simulink model "power_microgrid_LTE_DR"  (R2017b)
settings: Solver=ode23tb  StartTime=0.0  StopTime=7.5  FixedStep=1/(1000)  MaxStep=60  RelTol=1e-4
PreLoadFcn:
  | load('solar_load_data_24h.mat')
values from neighbouring files (symbols this model uses):
  HPD_1min = [1086.95652174 1079.71014493 1072.46376812 1065.2173913 1057.97101449 1050.72463768 1043.47826087 1036.23188406 1028.98550725 1021.73913043 1014.49275362 1007.24637681 ... (1441 elements, 1441x1)]    [HBD_1min.mat]
  HPT_1min = [0.01 0.02 0.03 0.04 0.05 0.06 0.07 0.08 0.09 0.1 0.11 0.12 ... (1441 elements, 1441x1)]    [HPT_1min.mat]    (also in MainTest.m = (0:7.5/1440:7.5)')
  SPD_1min = [0 0 0 0 0 0 0 0 0 0 0 0 ... (1441 elements, 1441x1)]    [SBD_1min.mat]
  SPT_1min = (0:7.5/1440:7.5)'    [MainTest.m]    (also in SPT_1min.mat = [0 60 120 180 240 300 360 420 480 540 600 660 ... (1441 elem)
undefined symbols (not defined in the file or in its folder): advanceLTEsim, advanceLTEsimulator, appLayer, entity, toAppLayer
libraries: powerlib x27
Description:
  | Copyright 2008-2017 The MathWorks, Inc.
settings Model: ModifiedByFormat=SPS  ExtModeTrigMode=oneshot  ExtModeArmWhenConnect=off  Creator=MathWorks  LastModifiedBy=SPS
settings SolverCC: InitialStep=1e-4  ZeroCrossAlgorithm=Adaptive
settings DataIOCC: SaveFormat=Array  SignalLoggingSaveFormat=ModelDataLogs  SaveOutput=off  SaveTime=off  SignalLoggingName=sigsOut
settings OptimizationCC: BooleanDataType=off  ExpressionDepthLimit=2147483647  InitFltsAndDblsToZero=on  LifeSpan=inf
settings DebuggingCC: AlgebraicLoopMsg=none  SaveWithParameterizedLinksMsg=none  UnderspecifiedInitializationDetection=Classic  MergeDetectMultiDrivingBlocksExec=none  SignalResolutionControl=TryResolveAllWithWarning  MultiTaskDSMMsg=warning  MultiTaskCondExecSysMsg=none  FcnCallInpInsideContextMsg=warning  AllowSymbolicDim=off  StateNameClashWarn=warning  SFUnexpectedBacktrackingDiag=warning  SFNoUnconditionalDefaultTransitionDiag=warning  SFExecutionAtInitializationDiag=none
settings HardwareCC: ProdBitPerPointer=32  ProdBitPerSizeT=32  ProdBitPerPtrDiffT=32  ProdLargestAtomicFloat=None  ProdIntDivRoundTo=Undefined  ProdEndianess=Unspecified  ProdWordSize=32  ProdHWDeviceType=32-bit Generic  TargetUnknown=on
settings ModelReferenceCC: PropagateSignalLabelsOutOfModel=off
settings RTWCC: Description=Generic Real-Time Target
settings CodeAppCC: StateflowObjectComments=on
settings GRTTargetCC: TargetFcnLib=ansi_tfl_tmw.mat  TargetLangStandard=C89/C90 (ANSI)  GeneratePreprocessorConditionals=Disable all  CombineOutputUpdateFcns=off  GRTInterface=on
settings ConfigComp: CovMetricSettings=dw  CovHtmlReporting=on  CovSaveCumulativeToWorkspaceVar=on  CovSaveSingleToWorkspaceVar=on  CovExternalEMLEnable=off  CovSFcnEnable=off
settings SimscapeCC: SimscapeNormalizeSystem=off

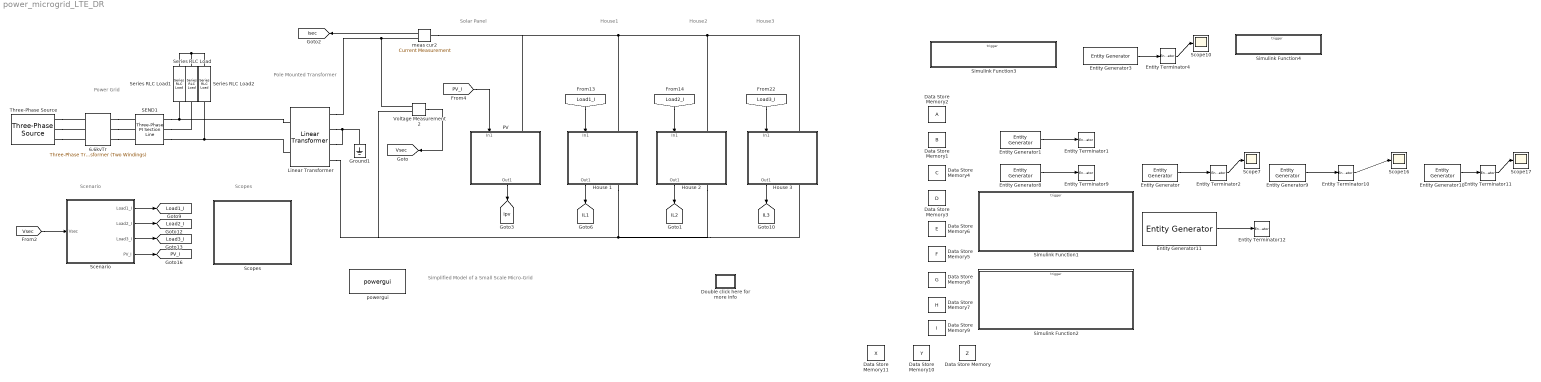
== system power_microgrid_LTE_DR ==
  note: Power Grid
  note: Pole Mounted
      | Transformer
  note: Solar Panel
  note: House1
  note: House2
  note: House3
  note: Scenario
  note: Scopes
  note: Simplified Model of a Small Scale Micro-Grid
  6.6kvTr : powerlib/Elements/Three-Phase Transformer (Two Windings)  Winding1Connection=Yg  Winding2Connection=Y  CoreType=Three single-phase transformers  SetSaturation=off  Hysteresis=off  DataFile='hysteresis'  SetInitialFlux=off  Measurements=None  UNITS=pu  NominalPower=[ 10e6 , 60 ]  Winding1=[ 66e3 , 0.002 , 0.08 ]  Winding2=[6.6e3 , 0.002 , 0.08 ]  Rm=500  Lm=500  L0=0.5  Saturation=[ 0,0 ; 0.0024,1.2 ; 1.0,1.52 ]  InitialFluxes=[ 0.8 , -0.8 , 0.7 ]  MoreParameters=off  BreakLoop=on  DataType=off  TransfoNumber=1
  Data Store Memory : DataStoreMemory  DataStoreName=Z  ReadBeforeWriteMsg=warning  WriteAfterWriteMsg=warning  WriteAfterReadMsg=warning  ShowAdditionalParam=off
  Data Store Memory1 : DataStoreMemory  DataStoreName=B  ReadBeforeWriteMsg=warning  WriteAfterWriteMsg=warning  WriteAfterReadMsg=warning  ShowAdditionalParam=off
  Data Store Memory10 : DataStoreMemory  DataStoreName=Y  ReadBeforeWriteMsg=warning  WriteAfterWriteMsg=warning  WriteAfterReadMsg=warning  ShowAdditionalParam=off
  Data Store Memory11 : DataStoreMemory  DataStoreName=X  ReadBeforeWriteMsg=warning  WriteAfterWriteMsg=warning  WriteAfterReadMsg=warning  ShowAdditionalParam=off
  Data Store Memory2 : DataStoreMemory  ReadBeforeWriteMsg=warning  WriteAfterWriteMsg=warning  WriteAfterReadMsg=warning  ShowAdditionalParam=off
  Data Store Memory3 : DataStoreMemory  DataStoreName=D  ReadBeforeWriteMsg=warning  WriteAfterWriteMsg=warning  WriteAfterReadMsg=warning  ShowAdditionalParam=off
  Data Store Memory4 : DataStoreMemory  DataStoreName=C  ReadBeforeWriteMsg=warning  WriteAfterWriteMsg=warning  WriteAfterReadMsg=warning  ShowAdditionalParam=off
  Data Store Memory5 : DataStoreMemory  DataStoreName=F  ReadBeforeWriteMsg=warning  WriteAfterWriteMsg=warning  WriteAfterReadMsg=warning  ShowAdditionalParam=off
  Data Store Memory6 : DataStoreMemory  DataStoreName=E  ReadBeforeWriteMsg=warning  WriteAfterWriteMsg=warning  WriteAfterReadMsg=warning  ShowAdditionalParam=off
  Data Store Memory7 : DataStoreMemory  DataStoreName=H  ReadBeforeWriteMsg=warning  WriteAfterWriteMsg=warning  WriteAfterReadMsg=warning  ShowAdditionalParam=off
  Data Store Memory8 : DataStoreMemory  DataStoreName=G  ReadBeforeWriteMsg=warning  WriteAfterWriteMsg=warning  WriteAfterReadMsg=warning  ShowAdditionalParam=off
  Data Store Memory9 : DataStoreMemory  DataStoreName=I  ReadBeforeWriteMsg=warning  WriteAfterWriteMsg=warning  WriteAfterReadMsg=warning  ShowAdditionalParam=off
  Double click here for more info : Subsystem
      settings: OpenFcn=showdemo(bdroot(gcb))
      mask Display: disp('?')
  Entity Generator : EntityGenerator  OutputPortMessageModes=m  Period=0.02  GenerateAction=|  AttributeName=nodeID|eventID|Demand  AttributeInitialValue=2|1|1  EntityType=Structured  EntityTypeName=LoadReport1
      | entity.Demand = ReadP();
      | toAppLayer(entity.nodeID,entity.eventID,entity.Demand,0);
  Entity Generator1 : EntityGenerator  OutputPortMessageModes=m  TimeSource=MATLAB action  IntergenerationTimeAction=dt = 0.02; %betarnd(4,4);  GenerateAction=toAppLayer(entity.NodeID,entity.eventID,0,0)  AttributeName=NodeID|eventID  AttributeInitialValue=7|1  EntityType=Structured  EntityTypeName=Forecast
  Entity Generator10 : EntityGenerator  OutputPortMessageModes=m  Period=0.02  GenerateAction=|  AttributeName=nodeID|eventID|Demand  AttributeInitialValue=4|1|1  EntityType=Structured  EntityTypeName=LoadReport3
      | entity.Demand = ReadP();
      | toAppLayer(entity.nodeID,entity.eventID,entity.Demand,0);
  Entity Generator11 : EntityGenerator  OutputPortMessageModes=m  Period=0.02  GenerateAction=|  AttributeName=nodeID|eventID|Psecondary  AttributeInitialValue=1|3|1  EntityType=Structured  EntityTypeName=PriceUpdate_SSPreading
      | entity.Psecondary = ReadPss();
      | toAppLayer(entity.nodeID,entity.eventID,entity.Psecondary,0);
  Entity Generator3 : EntityGenerator  OutputPortMessageModes=m  Period=0.001  GenerateEntityAtSimulationStart=off  GenerateAction=advanceLTEsimulator(entity.data)  AttributeName=data  EntityType=Structured  EntityTypeName=TTIadvance
  Entity Generator8 : EntityGenerator  OutputPortMessageModes=m  TimeSource=MATLAB action  IntergenerationTimeAction=dt = 0.016; %betarnd(4,4);  GenerateAction=toAppLayer(entity.NodeID,entity.eventID,0,0);  AttributeName=NodeID|eventID|phase  AttributeInitialValue=5|1|0  EntityType=Structured  EntityTypeName=PhaseReport
  Entity Generator9 : EntityGenerator  OutputPortMessageModes=m  Period=0.02  GenerateAction=|  AttributeName=nodeID|eventID|Demand  AttributeInitialValue=3|1|1  EntityType=Structured  EntityTypeName=LoadReport2
      | entity.Demand = ReadP();
      | toAppLayer(entity.nodeID,entity.eventID,entity.Demand,0);
  Entity Terminator1 : EntityTerminator  InputPortMessageModes=m
  Entity Terminator{2,4,10..11} (4 alike) : EntityTerminator  InputPortMessageModes=m  NumberEntitiesArrived=on
      settings: OutputPortMap=o0
  Entity Terminator12 : EntityTerminator  InputPortMessageModes=m
  Entity Terminator9 : EntityTerminator  InputPortMessageModes=m
  Ground1 : powerlib/Elements/Ground  LConnTagsString=a
  House 1 : Subsystem
      mask Display: image(imread('house.jpg'))
  House 2 : Subsystem
      mask Display: image(imread('house.jpg'))
  House 3 : Subsystem
      mask Display: image(imread('house.jpg'))
  Linear Transformer : powerlib/Elements/Linear Transformer  UNITS=pu  NominalPower=[75e3 60]  winding1=[ 6600 0.00005 0.0002 ]  winding2=[ 100 0.00005 0.0002 ]  ThreeWindings=on  winding3=[ 100 0.00005 0.0002 ]  RmLm=[ 50 50 ]  Measurements=None  DataType=off
  PV : Subsystem
      mask Display: image(imread('pv.jpg'))
  SEND1 : powerlib/Elements/Three-Phase PI Section Line  LConnTagsString=a|b|c  RConnTagsString=A|B|C  Frequency=60  Resistances=[ 0.01273 0.3864]  Inductances="[ 0.9337e-3  4.1264e-3]"  Capacitances=[12.74e-9 7.751e-9]  Length=1
      settings: SourceProductName=Simscape Power Systems
  Scenario : Subsystem
  Scope{7,10,16..17} (4 alike) : Scope
  Scopes : Subsystem
  Series RLC Load : powerlib/Elements/Series RLC Load  LConnTagsString=a  RConnTagsString=__new0  NominalVoltage=1000  NominalFrequency=60  ActivePower=10e3  InductivePower=100  CapacitivePower=100  Setx0=off  InitialVoltage=0  SetiL0=off  InitialCurrent=0  Measurements=None  LoadType=constant Z
  Series RLC Load1 : powerlib/Elements/Series RLC Load  LConnTagsString=a  RConnTagsString=__new0  NominalVoltage=1000  NominalFrequency=60  ActivePower=100e3  InductivePower=100  CapacitivePower=100  Setx0=off  InitialVoltage=0  SetiL0=off  InitialCurrent=0  Measurements=None  LoadType=constant Z
  Series RLC Load2 : powerlib/Elements/Series RLC Load  LConnTagsString=a  RConnTagsString=__new0  NominalVoltage=1000  NominalFrequency=60  ActivePower=10e3  InductivePower=100  CapacitivePower=100  Setx0=off  InitialVoltage=0  SetiL0=off  InitialCurrent=0  Measurements=None  LoadType=constant Z
  Simulink Function1 : Subsystem  TreatAsAtomicUnit=on
  Simulink Function2 : Subsystem  TreatAsAtomicUnit=on
  Simulink Function3 : Subsystem  TreatAsAtomicUnit=on
  Simulink Function4 : Subsystem  TreatAsAtomicUnit=on
  Three-Phase Source : powerlib/Electrical Sources/Three-Phase Source  InternalConnection=Yg  VoltagePhases=off  Voltage=66e3  PhaseAngle=0  Voltage_phases=[25e3 25e3 25e3]/sqrt(3)  PhaseAngles_phases=[0 -120 +120]  Frequency=60  NonIdealSource=on  SpecifyImpedance=on  Resistance=0.8929  Inductance=16.58e-3  ShortCircuitLevel=100e6  BaseVoltage=25e3  XRratio=7  BusType=swing  Pref=0  Qref=0  Prefabc=[10e3, 10e3, 10e3]  Qrefabc=[0, 0, 0]  Qmin=-inf  Qmax=inf
  Voltage Measurement2 : powerlib/Measurements/Voltage Measurement  PhasorSimulation=on  OutputType=Complex  PSBequivalent=0
  meas cur2 : powerlib/Measurements/Current Measurement  PhasorSimulation=on  OutputType=Complex  PSBequivalent=0
  powergui : powerlib/powergui  SimulationMode=Phasor  SampleTime=1/60/100  frequency=60  Iterations=50  frequencyindice=60  Pbase=100e6  ErrMax=1e-4  UnitsV=kV  UnitsW=MW  buscounter=0  FunctionMessages=off  echomessages=off  EnableUseOfTLC=off  CurrentSourceSwitches=off  DisableSnubberDevices=off  DisableRonSwitches=off  DisableVfSwitches=off  DisplayEquations=off  SolverType=Tustin  Interpol=off  ExternalGateDelay=off  methode=off  Ts=0  x0status=blocks  SPID=off  SwTol=0  HookPort=off  RestoreLinks=warning  ResistiveCurrentMeasurement=off  Frange=[0:2:500]  Ylog=off  Xlog=on  ShowGrid=off  save=off  variable=ZData  structure=0  ZoomFFT=on  StartTime=0.0  cycles=1  DisplayStyle=1  fundamental=60  FreqAxis=off  MaxFrequency=1000  frequencyindicesteady=1  RmsSteady=1  display=off
  tag scope: IL1=global, IL2=global, IL3=global, Ipv=global, Isec=global, Load1_I=global, Load2_I=global, Load3_I=global, PV_I=global, Vsec=global
  wires:
  House 2/1(Out1) -> [IL2]
  House 1/1(Out1) -> [IL1]
  House 3/1(Out1) -> [IL3]
  [Load2_I] -> House 2/1(In1)
  [Load3_I] -> House 3/1(In1)
  PV/1(Out1) -> [Ipv]
  [Vsec] -> Scenario/1(Vsec)
  [Load1_I] -> House 1/1(In1)
  [PV_I] -> PV/1(In1)
  Entity Terminator4/1 -> Scope10/1
  Voltage Measurement2/1 -> [Vsec]
  meas cur2/1 -> [Isec]
  Entity Terminator2/1 -> Scope7/1
  Entity Terminator10/1 -> Scope16/1
  Entity Terminator11/1 -> Scope17/1
  Scenario/4(PV_I) -> [PV_I]
  Scenario/3(Load3_I) -> [Load3_I]
  Scenario/2(Load2_I) -> [Load2_I]
  Scenario/1(Load1_I) -> [Load1_I]
  Entity Generator11/1 -> Entity Terminator12/1
  Entity Generator/1 -> Entity Terminator2/1
  Entity Generator8/1 -> Entity Terminator9/1
  Entity Generator9/1 -> Entity Terminator10/1
  Entity Generator10/1 -> Entity Terminator11/1
  Entity Generator3/1 -> Entity Terminator4/1
  Entity Generator1/1 -> Entity Terminator1/1
  connections:
  SEND1/RConn3 -- Linear Transformer/LConn2 -- Series RLC Load2/RConn1
  6.6kvTr/RConn2 -- SEND1/LConn2
  6.6kvTr/RConn1 -- SEND1/LConn1
  Three-Phase Source/RConn1 -- 6.6kvTr/LConn1
  Three-Phase Source/RConn3 -- 6.6kvTr/LConn3
  6.6kvTr/RConn3 -- SEND1/LConn3
  Ground1/LConn1 -- Linear Transformer/RConn3 -- Linear Transformer/RConn2
  Three-Phase Source/RConn2 -- 6.6kvTr/LConn2
  SEND1/RConn2 -- Series RLC Load/RConn1
  Series RLC Load1/LConn1 -- Series RLC Load/LConn1 -- Series RLC Load2/LConn1
  SEND1/RConn1 -- Linear Transformer/LConn1 -- Series RLC Load1/RConn1
  Linear Transformer/RConn1 -- Voltage Measurement2/LConn1 -- meas cur2/RConn1
  House 2/RConn1 -- House 3/RConn1 -- Linear Transformer/RConn4 -- Voltage Measurement2/LConn2 -- House 1/RConn1
  House 1/LConn1 -- PV/LConn1 -- meas cur2/LConn1 -- House 2/LConn1 -- House 3/LConn1

== system power_microgrid_LTE_DR/Double click here for more info ==

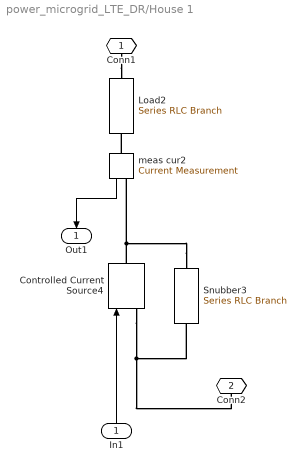
== system power_microgrid_LTE_DR/House 1 ==
  In1 : Inport
  Controlled Current Source4 : powerlib/Electrical Sources/Controlled Current Source  Initialize=on  Source_Type=AC  Amplitude=0  Phase=30  Frequency=60  Measurements=None
  Load2 : powerlib/Elements/Series RLC Branch  LConnTagsString=__new0  RConnTagsString=__new0  BranchType=R  Resistance=16  Inductance=1e-3  SetiL0=off  InitialCurrent=0  Capacitance=1e-6  Setx0=off  InitialVoltage=0  Measurements=None
  Snubber3 : powerlib/Elements/Series RLC Branch  LConnTagsString=__new0  RConnTagsString=__new0  BranchType=R  Resistance=1e6  Inductance=1e-3  SetiL0=off  InitialCurrent=0  Capacitance=1e-6  Setx0=off  InitialVoltage=0  Measurements=None
  meas cur2 : powerlib/Measurements/Current Measurement  PhasorSimulation=on  OutputType=Complex  PSBequivalent=0
  Conn1 : PMIOPort  Port=1  Side=Left
  Conn2 : PMIOPort  Port=2  Side=Right
  Out1 : Outport
  wires:
  In1/1 -> Controlled Current Source4/1
  meas cur2/1 -> Out1/1
  connections:
  Conn1/RConn1 -- Load2/LConn1
  meas cur2/LConn1 -- Load2/RConn1
  Snubber3/LConn1 -- meas cur2/RConn1 -- Controlled Current Source4/RConn1
  Snubber3/RConn1 -- Conn2/RConn1 -- Controlled Current Source4/LConn1

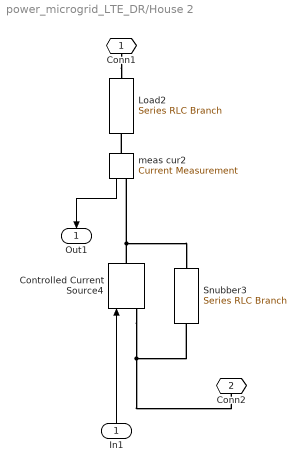
== system power_microgrid_LTE_DR/House 2 ==
  In1 : Inport
  Controlled Current Source4 : powerlib/Electrical Sources/Controlled Current Source  Initialize=on  Source_Type=AC  Amplitude=0  Phase=30  Frequency=60  Measurements=None
  Load2 : powerlib/Elements/Series RLC Branch  LConnTagsString=__new0  RConnTagsString=__new0  BranchType=R  Resistance=16  Inductance=1e-3  SetiL0=off  InitialCurrent=0  Capacitance=1e-6  Setx0=off  InitialVoltage=0  Measurements=None
  Snubber3 : powerlib/Elements/Series RLC Branch  LConnTagsString=__new0  RConnTagsString=__new0  BranchType=R  Resistance=1e6  Inductance=1e-3  SetiL0=off  InitialCurrent=0  Capacitance=1e-6  Setx0=off  InitialVoltage=0  Measurements=None
  meas cur2 : powerlib/Measurements/Current Measurement  PhasorSimulation=on  OutputType=Complex  PSBequivalent=0
  Conn1 : PMIOPort  Port=1  Side=Left
  Conn2 : PMIOPort  Port=2  Side=Right
  Out1 : Outport
  wires:
  meas cur2/1 -> Out1/1
  In1/1 -> Controlled Current Source4/1
  connections:
  Controlled Current Source4/LConn1 -- Conn2/RConn1 -- Snubber3/RConn1
  Controlled Current Source4/RConn1 -- meas cur2/RConn1 -- Snubber3/LConn1
  meas cur2/LConn1 -- Load2/RConn1
  Conn1/RConn1 -- Load2/LConn1

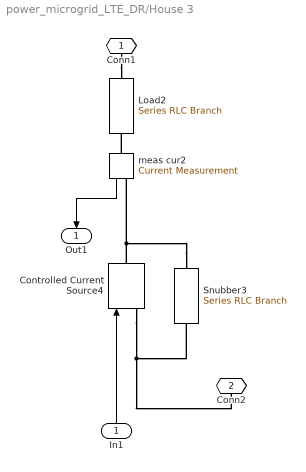
== system power_microgrid_LTE_DR/House 3 ==
  In1 : Inport
  Controlled Current Source4 : powerlib/Electrical Sources/Controlled Current Source  Initialize=on  Source_Type=AC  Amplitude=0  Phase=30  Frequency=60  Measurements=None
  Load2 : powerlib/Elements/Series RLC Branch  LConnTagsString=__new0  RConnTagsString=__new0  BranchType=R  Resistance=16  Inductance=1e-3  SetiL0=off  InitialCurrent=0  Capacitance=1e-6  Setx0=off  InitialVoltage=0  Measurements=None
  Snubber3 : powerlib/Elements/Series RLC Branch  LConnTagsString=__new0  RConnTagsString=__new0  BranchType=R  Resistance=1e6  Inductance=1e-3  SetiL0=off  InitialCurrent=0  Capacitance=1e-6  Setx0=off  InitialVoltage=0  Measurements=None
  meas cur2 : powerlib/Measurements/Current Measurement  PhasorSimulation=on  OutputType=Complex  PSBequivalent=0
  Conn1 : PMIOPort  Port=1  Side=Left
  Conn2 : PMIOPort  Port=2  Side=Right
  Out1 : Outport
  wires:
  In1/1 -> Controlled Current Source4/1
  meas cur2/1 -> Out1/1
  connections:
  Conn1/RConn1 -- Load2/LConn1
  meas cur2/LConn1 -- Load2/RConn1
  Snubber3/LConn1 -- meas cur2/RConn1 -- Controlled Current Source4/RConn1
  Snubber3/RConn1 -- Conn2/RConn1 -- Controlled Current Source4/LConn1

== system power_microgrid_LTE_DR/PV ==
  In1 : Inport
  Controlled Current Source : powerlib/Electrical Sources/Controlled Current Source  Initialize=on  Source_Type=AC  Amplitude=0  Phase=30  Frequency=60  Measurements=None
  Ground2 : powerlib/Elements/Ground  LConnTagsString=a
  Snubber1 : powerlib/Elements/Series RLC Branch  LConnTagsString=__new0  RConnTagsString=__new0  BranchType=R  Resistance=1e6  Inductance=1e-3  SetiL0=off  InitialCurrent=0  Capacitance=1e-6  Setx0=off  InitialVoltage=0  Measurements=None
  meas cur3 : powerlib/Measurements/Current Measurement  PhasorSimulation=on  OutputType=Complex  PSBequivalent=0
  Conn1 : PMIOPort  Port=1  Side=Left
  Out1 : Outport
  wires:
  meas cur3/1 -> Out1/1
  In1/1 -> Controlled Current Source/1
  connections:
  Ground2/LConn1 -- Controlled Current Source/LConn1 -- Snubber1/RConn1
  Snubber1/LConn1 -- Controlled Current Source/RConn1 -- meas cur3/LConn1
  Conn1/RConn1 -- meas cur3/RConn1

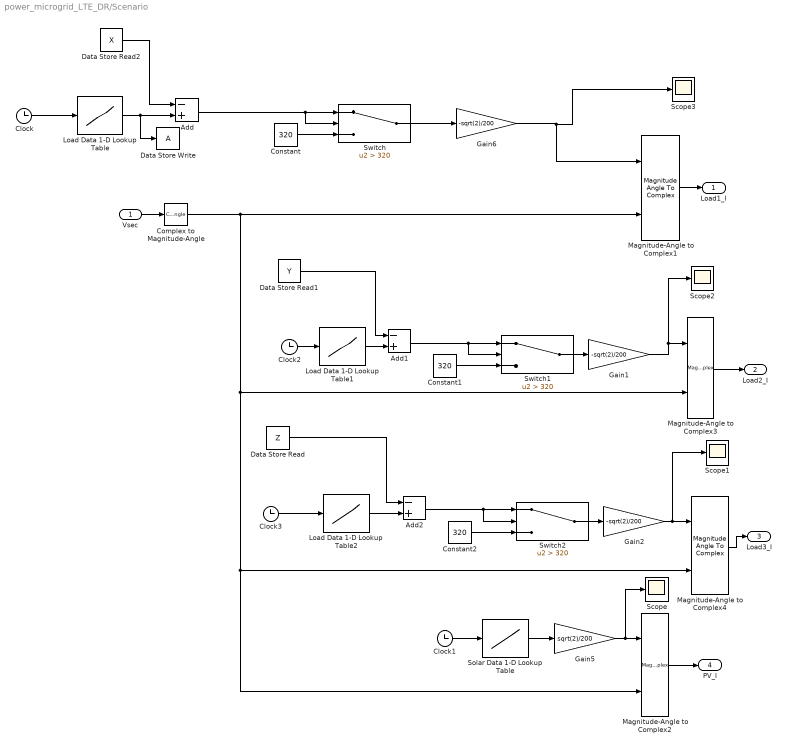
== system power_microgrid_LTE_DR/Scenario ==
  Vsec : Inport
  Add : Sum  Inputs=-+
  Add1 : Sum  Inputs=-+
  Add2 : Sum  Inputs=-+
  Clock{,1..3} (4 alike) : Clock
  Complex to Magnitude-Angle : ComplexToMagnitudeAngle  Output=Angle
  Constant : Constant  Value=320
  Constant1 : Constant  Value=320
  Constant2 : Constant  Value=320
  Data Store Read : DataStoreRead  DataStoreName=Z
  Data Store Read1 : DataStoreRead  DataStoreName=Y
  Data Store Read2 : DataStoreRead  DataStoreName=X
  Data Store Write : DataStoreWrite
  Gain1 : Gain  Gain=-sqrt(2)/200
  Gain2 : Gain  Gain=-sqrt(2)/200
  Gain5 : Gain  Gain=sqrt(2)/200
  Gain6 : Gain  Gain=-sqrt(2)/200
  Load Data 1-D Lookup Table : Lookup_n-D  NumberOfTableDimensions=1  BreakpointsForDimension1=HPT_1min  Table=HPD_1min  InternalRulePriority=Speed  RndMeth=Simplest  InputSameDT=on
  Load Data 1-D Lookup Table1 : Lookup_n-D  NumberOfTableDimensions=1  BreakpointsForDimension1=HPT_1min  Table=HPD_1min  InternalRulePriority=Speed  RndMeth=Simplest  InputSameDT=on
  Load Data 1-D Lookup Table2 : Lookup_n-D  NumberOfTableDimensions=1  BreakpointsForDimension1=HPT_1min  Table=HPD_1min  InternalRulePriority=Speed  RndMeth=Simplest  InputSameDT=on
  Magnitude-Angle to Complex{1..4} (4 alike) : MagnitudeAngleToComplex
  Scope{,1..3} (4 alike) : Scope
  Solar Data 1-D Lookup Table : Lookup_n-D  NumberOfTableDimensions=1  BreakpointsForDimension1=SPT_1min  Table=SPD_1min  InternalRulePriority=Speed  RndMeth=Simplest  InputSameDT=on
  Switch : Switch  Criteria=u2 > Threshold  Threshold=320
  Switch1 : Switch  Criteria=u2 > Threshold  Threshold=320
  Switch2 : Switch  Criteria=u2 > Threshold  Threshold=320
  Load1_I : Outport
  Load2_I : Outport  Port=2
  Load3_I : Outport  Port=3
  PV_I : Outport  Port=4
  wires:
  Magnitude-Angle to Complex4/1 -> Load3_I/1
  Magnitude-Angle to Complex2/1 -> PV_I/1
  Load Data 1-D Lookup Table/1 -> Data Store Write/1, Add/2
  Solar Data 1-D Lookup Table/1 -> Gain5/1
  Clock1/1 -> Solar Data 1-D Lookup Table/1
  Clock3/1 -> Load Data 1-D Lookup Table2/1
  Gain2/1 -> Scope1/1, Magnitude-Angle to Complex4/1
  Magnitude-Angle to Complex1/1 -> Load1_I/1
  Gain5/1 -> Scope/1, Magnitude-Angle to Complex2/1
  Complex to Magnitude-Angle/1 -> Magnitude-Angle to Complex1/2, Magnitude-Angle to Complex4/2, Magnitude-Angle to Complex2/2, Magnitude-Angle to Complex3/2
  Magnitude-Angle to Complex3/1 -> Load2_I/1
  Vsec/1 -> Complex to Magnitude-Angle/1
  Clock2/1 -> Load Data 1-D Lookup Table1/1
  Clock/1 -> Load Data 1-D Lookup Table/1
  Load Data 1-D Lookup Table1/1 -> Add1/2
  Load Data 1-D Lookup Table2/1 -> Add2/2
  Data Store Read2/1 -> Add/1
  Data Store Read1/1 -> Add1/1
  Data Store Read/1 -> Add2/1
  Add/1 -> Switch/2, Switch/1
  Constant/1 -> Switch/3
  Switch/1 -> Gain6/1
  Add1/1 -> Switch1/2, Switch1/1
  Constant1/1 -> Switch1/3
  Gain6/1 -> Scope3/1, Magnitude-Angle to Complex1/1
  Switch1/1 -> Gain1/1
  Gain1/1 -> Scope2/1, Magnitude-Angle to Complex3/1
  Constant2/1 -> Switch2/3
  Add2/1 -> Switch2/2, Switch2/1
  Switch2/1 -> Gain2/1

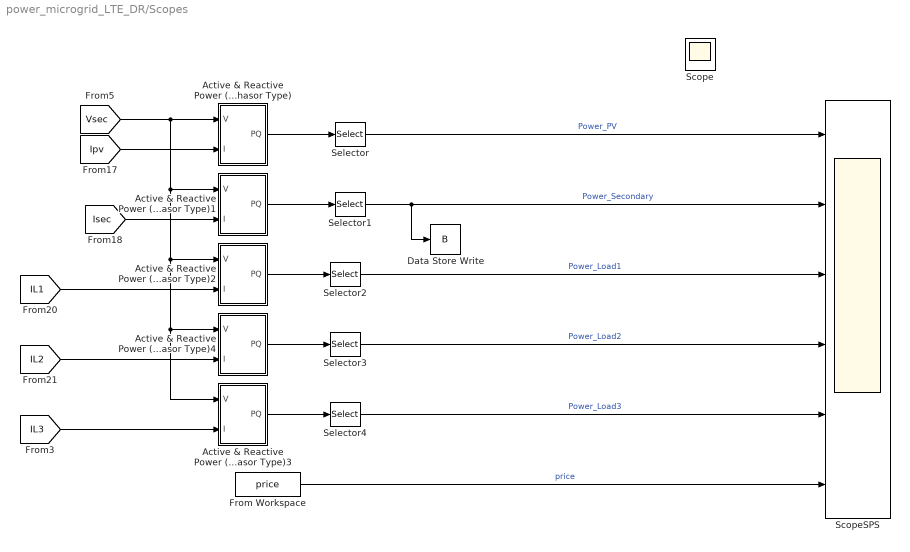
== system power_microgrid_LTE_DR/Scopes ==
  Active & Reactive Power (Phasor Type) : Subsystem  DialogController=POWERSYS.PowerSysDialog  mask(Active & Reactive Power (Phasor Type)){}
      mask help: Active & Reactive Power (Phasor Type)
      mask init:
      | power_initmask();
      mask Help: This block is part of a subset of blocks in the Extras library that does not have documentation associated with it, other than the block mask description.
      mask Display: disp('')
  Active & Reactive Power (Phasor Type)1 : Subsystem  DialogController=POWERSYS.PowerSysDialog  mask(Active & Reactive Power (Phasor Type)){}
      mask help: Active & Reactive Power (Phasor Type)
      mask init:
      | power_initmask();
      mask Help: This block is part of a subset of blocks in the Extras library that does not have documentation associated with it, other than the block mask description.
      mask Display: disp('')
  Active & Reactive Power (Phasor Type)2 : Subsystem  DialogController=POWERSYS.PowerSysDialog  mask(Active & Reactive Power (Phasor Type)){}
      mask help: Active & Reactive Power (Phasor Type)
      mask init:
      | power_initmask();
      mask Help: This block is part of a subset of blocks in the Extras library that does not have documentation associated with it, other than the block mask description.
      mask Display: disp('')
  Active & Reactive Power (Phasor Type)3 : Subsystem  DialogController=POWERSYS.PowerSysDialog  mask(Active & Reactive Power (Phasor Type)){}
      mask help: Active & Reactive Power (Phasor Type)
      mask init:
      | power_initmask();
      mask Help: This block is part of a subset of blocks in the Extras library that does not have documentation associated with it, other than the block mask description.
      mask Display: disp('')
  Active & Reactive Power (Phasor Type)4 : Subsystem  DialogController=POWERSYS.PowerSysDialog  mask(Active & Reactive Power (Phasor Type)){}
      mask help: Active & Reactive Power (Phasor Type)
      mask init:
      | power_initmask();
      mask Help: This block is part of a subset of blocks in the Extras library that does not have documentation associated with it, other than the block mask description.
      mask Display: disp('')
  Data Store Write : DataStoreWrite  DataStoreName=B
  From Workspace : FromWorkspace  VariableName=price  SampleTime=0
  Scope : Scope
  ScopeSPS : Scope  NumInputPorts=6
  Selector{,1..4} (5 alike) : Selector  InputPortWidth=2  IndexOptions=Index vector (dialog)  Indices=1  OutputSizes=1
  wires:
  Selector3/1 -> ScopeSPS/4  "Power_Load2"
  From Workspace/1 -> ScopeSPS/6  "price"
  [Ipv] -> Active & Reactive Power (Phasor Type)/2(I)
  Active & Reactive Power (Phasor Type)2/1(PQ) -> Selector2/1
  Active & Reactive Power (Phasor Type)1/1(PQ) -> Selector1/1
  Selector/1 -> ScopeSPS/1  "Power_PV"
  Active & Reactive Power (Phasor Type)/1(PQ) -> Selector/1
  [Vsec] -> Active & Reactive Power (Phasor Type)3/1(V), Active & Reactive Power (Phasor Type)4/1(V), Active & Reactive Power (Phasor Type)2/1(V), Active & Reactive Power (Phasor Type)1/1(V), Active & Reactive Power (Phasor Type)/1(V)
  [IL2] -> Active & Reactive Power (Phasor Type)4/2(I)
  Selector1/1 -> Data Store Write/1, ScopeSPS/2  "Power_Secondary"
  Active & Reactive Power (Phasor Type)4/1(PQ) -> Selector3/1
  [IL3] -> Active & Reactive Power (Phasor Type)3/2(I)
  [IL1] -> Active & Reactive Power (Phasor Type)2/2(I)
  Active & Reactive Power (Phasor Type)3/1(PQ) -> Selector4/1
  Selector2/1 -> ScopeSPS/3  "Power_Load1"
  Selector4/1 -> ScopeSPS/5  "Power_Load3"
  [Isec] -> Active & Reactive Power (Phasor Type)1/2(I)

== system power_microgrid_LTE_DR/Simulink Function1 ==
  ReadP : TriggerPort  TriggerType=function-call  IsSimulinkFunction=on  FunctionName=ReadP  FunctionVisibility=scoped  VariantControl=(inherit)
  Data Store Read : DataStoreRead
  P : ArgOut  ArgumentName=P
  wires:
  Data Store Read/1 -> P/1

== system power_microgrid_LTE_DR/Simulink Function2 ==
  ReadPss : TriggerPort  TriggerType=function-call  IsSimulinkFunction=on  FunctionName=ReadPss  FunctionVisibility=scoped  VariantControl=(inherit)
  Data Store Read : DataStoreRead  DataStoreName=B
  P : ArgOut  ArgumentName=P
  wires:
  Data Store Read/1 -> P/1

== system power_microgrid_LTE_DR/Simulink Function3 ==
  toAppLayer : TriggerPort  TriggerType=function-call  IsSimulinkFunction=on  FunctionName=toAppLayer  FunctionVisibility=scoped  VariantControl=(inherit)
  Interpreted MATLAB Function : MATLABFcn  MATLABFcn=appLayer(u)  OutputDimensions=0
  Mux : Mux
  NodeID : ArgIn  DisableCoverage=on  ArgumentName=NodeID
  eventID : ArgIn  Port=2  ArgumentName=eventID
  reading1 : ArgIn  Port=3  ArgumentName=reading1
  reading2 : ArgIn  Port=4  ArgumentName=reading2
  wires:
  Mux/1 -> Interpreted MATLAB Function/1
  eventID/1 -> Mux/2
  NodeID/1 -> Mux/1
  reading1/1 -> Mux/3
  reading2/1 -> Mux/4

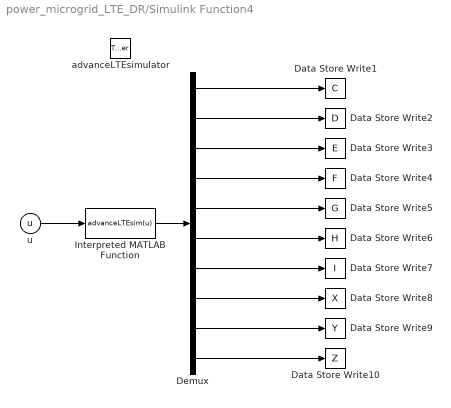
== system power_microgrid_LTE_DR/Simulink Function4 ==
  advanceLTEsimulator : TriggerPort  TriggerType=function-call  IsSimulinkFunction=on  FunctionName=advanceLTEsimulator  FunctionVisibility=scoped  VariantControl=(inherit)
  Data Store Write1 : DataStoreWrite  DataStoreName=C
  Data Store Write10 : DataStoreWrite  DataStoreName=Z
  Data Store Write2 : DataStoreWrite  DataStoreName=D
  Data Store Write3 : DataStoreWrite  DataStoreName=E
  Data Store Write4 : DataStoreWrite  DataStoreName=F
  Data Store Write5 : DataStoreWrite  DataStoreName=G
  Data Store Write6 : DataStoreWrite  DataStoreName=H
  Data Store Write7 : DataStoreWrite  DataStoreName=I
  Data Store Write8 : DataStoreWrite  DataStoreName=X
  Data Store Write9 : DataStoreWrite  DataStoreName=Y
  Demux : Demux  Outputs=10
  Interpreted MATLAB Function : MATLABFcn  MATLABFcn=advanceLTEsim(u)
  u : ArgIn  ArgumentName=u
  wires:
  Interpreted MATLAB Function/1 -> Demux/1
  Demux/1 -> Data Store Write1/1
  Demux/2 -> Data Store Write2/1
  Demux/3 -> Data Store Write3/1
  Demux/4 -> Data Store Write4/1
  Demux/5 -> Data Store Write5/1
  Demux/6 -> Data Store Write6/1
  Demux/7 -> Data Store Write7/1
  u/1 -> Interpreted MATLAB Function/1
  Demux/8 -> Data Store Write8/1
  Demux/9 -> Data Store Write9/1
  Demux/10 -> Data Store Write10/1

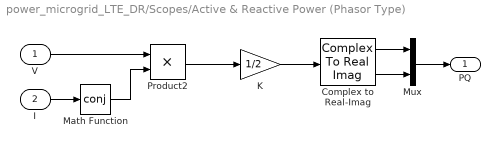
== system power_microgrid_LTE_DR/Scopes/Active & Reactive Power (Phasor Type) ==
  V : Inport
  I : Inport  Port=2
  Complex to Real-Imag : ComplexToRealImag
  K : Gain  Gain=1/2  SaturateOnIntegerOverflow=on  OutDataTypeStr=Inherit: Same as input  ParamDataTypeStr=Inherit: Same as input
  Math Function : Math  Operator=conj  SaturateOnIntegerOverflow=on
  Mux : Mux  Inputs=2
  Product2 : Product  SaturateOnIntegerOverflow=on  InputSameDT=on  OutDataTypeStr=Inherit: Same as first input
  PQ : Outport
  wires:
  Mux/1 -> PQ/1
  Complex to Real-Imag/2 -> Mux/2
  Complex to Real-Imag/1 -> Mux/1
  V/1 -> Product2/1
  Math Function/1 -> Product2/2
  Product2/1 -> K/1
  K/1 -> Complex to Real-Imag/1
  I/1 -> Math Function/1

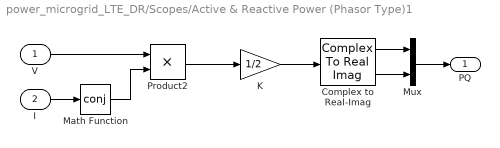
== system power_microgrid_LTE_DR/Scopes/Active & Reactive Power (Phasor Type)1 ==
  V : Inport
  I : Inport  Port=2
  Complex to Real-Imag : ComplexToRealImag
  K : Gain  Gain=1/2  SaturateOnIntegerOverflow=on  OutDataTypeStr=Inherit: Same as input  ParamDataTypeStr=Inherit: Same as input
  Math Function : Math  Operator=conj  SaturateOnIntegerOverflow=on
  Mux : Mux  Inputs=2
  Product2 : Product  SaturateOnIntegerOverflow=on  InputSameDT=on  OutDataTypeStr=Inherit: Same as first input
  PQ : Outport
  wires:
  Mux/1 -> PQ/1
  Complex to Real-Imag/2 -> Mux/2
  Complex to Real-Imag/1 -> Mux/1
  V/1 -> Product2/1
  Math Function/1 -> Product2/2
  Product2/1 -> K/1
  K/1 -> Complex to Real-Imag/1
  I/1 -> Math Function/1

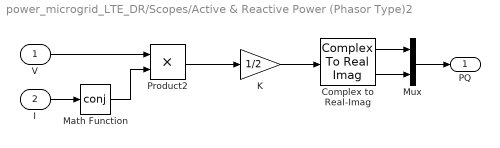
== system power_microgrid_LTE_DR/Scopes/Active & Reactive Power (Phasor Type)2 ==
  V : Inport
  I : Inport  Port=2
  Complex to Real-Imag : ComplexToRealImag
  K : Gain  Gain=1/2  SaturateOnIntegerOverflow=on  OutDataTypeStr=Inherit: Same as input  ParamDataTypeStr=Inherit: Same as input
  Math Function : Math  Operator=conj  SaturateOnIntegerOverflow=on
  Mux : Mux  Inputs=2
  Product2 : Product  SaturateOnIntegerOverflow=on  InputSameDT=on  OutDataTypeStr=Inherit: Same as first input
  PQ : Outport
  wires:
  Mux/1 -> PQ/1
  Complex to Real-Imag/2 -> Mux/2
  Complex to Real-Imag/1 -> Mux/1
  V/1 -> Product2/1
  Math Function/1 -> Product2/2
  Product2/1 -> K/1
  K/1 -> Complex to Real-Imag/1
  I/1 -> Math Function/1

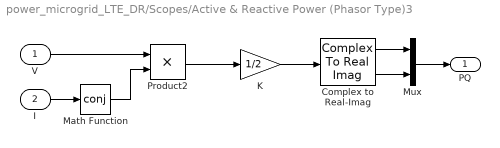
== system power_microgrid_LTE_DR/Scopes/Active & Reactive Power (Phasor Type)3 ==
  V : Inport
  I : Inport  Port=2
  Complex to Real-Imag : ComplexToRealImag
  K : Gain  Gain=1/2  SaturateOnIntegerOverflow=on  OutDataTypeStr=Inherit: Same as input  ParamDataTypeStr=Inherit: Same as input
  Math Function : Math  Operator=conj  SaturateOnIntegerOverflow=on
  Mux : Mux  Inputs=2
  Product2 : Product  SaturateOnIntegerOverflow=on  InputSameDT=on  OutDataTypeStr=Inherit: Same as first input
  PQ : Outport
  wires:
  Mux/1 -> PQ/1
  Complex to Real-Imag/2 -> Mux/2
  Complex to Real-Imag/1 -> Mux/1
  V/1 -> Product2/1
  Math Function/1 -> Product2/2
  Product2/1 -> K/1
  K/1 -> Complex to Real-Imag/1
  I/1 -> Math Function/1

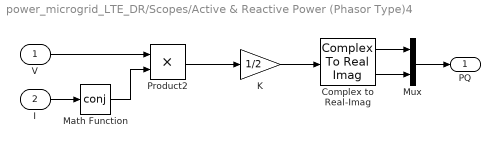
== system power_microgrid_LTE_DR/Scopes/Active & Reactive Power (Phasor Type)4 ==
  V : Inport
  I : Inport  Port=2
  Complex to Real-Imag : ComplexToRealImag
  K : Gain  Gain=1/2  SaturateOnIntegerOverflow=on  OutDataTypeStr=Inherit: Same as input  ParamDataTypeStr=Inherit: Same as input
  Math Function : Math  Operator=conj  SaturateOnIntegerOverflow=on
  Mux : Mux  Inputs=2
  Product2 : Product  SaturateOnIntegerOverflow=on  InputSameDT=on  OutDataTypeStr=Inherit: Same as first input
  PQ : Outport
  wires:
  Mux/1 -> PQ/1
  Complex to Real-Imag/2 -> Mux/2
  Complex to Real-Imag/1 -> Mux/1
  V/1 -> Product2/1
  Math Function/1 -> Product2/2
  Product2/1 -> K/1
  K/1 -> Complex to Real-Imag/1
  I/1 -> Math Function/1
